simulink library "basic_THB"  (R2016b)
settings: Solver=ode45  StartTime=0.0  StopTime=10.0  RelTol=1e-3  EnableMultiTasking=on
undefined symbols (not defined in the file): Water
settings Model: Creator=lena.frank  LastModifiedBy=awohlfei
settings DataIOCC: LimitDataPoints=on  SaveFormat=Array  SignalLoggingSaveFormat=ModelDataLogs
settings OptimizationCC: ExpressionDepthLimit=2147483647  LifeSpan=inf
settings DebuggingCC: UnderspecifiedInitializationDetection=Classic  MergeDetectMultiDrivingBlocksExec=none  SolverPrmCheckMsg=warning  FcnCallInpInsideContextMsg=warning  StateNameClashWarn=warning  SFUnexpectedBacktrackingDiag=warning  SFNoUnconditionalDefaultTransitionDiag=warning  SFExecutionAtInitializationDiag=none
settings HardwareCC: ProdBitPerPointer=32  ProdBitPerSizeT=32  ProdBitPerPtrDiffT=32  ProdLargestAtomicFloat=None  ProdIntDivRoundTo=Undefined  ProdEndianess=Unspecified  ProdWordSize=32  ProdHWDeviceType=32-bit Generic
settings ModelReferenceCC: PropagateSignalLabelsOutOfModel=off
settings GRTTargetCC: TargetLangStandard=C89/C90 (ANSI)  GeneratePreprocessorConditionals=Disable all  CombineOutputUpdateFcns=off  GRTInterface=on
settings ConfigComp: CovMetricSettings=dw  CovHtmlReporting=on  CovSaveCumulativeToWorkspaceVar=on  CovSaveSingleToWorkspaceVar=on  CovExternalEMLEnable=off

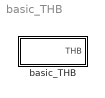
== system basic_THB ==
  basic_THB : Subsystem  InitFcn=load('THB.mat');  mask(basic THB){t=20, mdot=0, p=1e5, ID=Pressure Drop from Massflow, fluid=Water, mix=0, mix2=0, mix3=0, dia=0.02, hgt=0}
      mask prompts: t "temperature [°C]"; mdot "massflow [kg/s]"; p "pressure [Pa]"; ID "ID for pressure drop calculation"; mix "fluid mixture [0..1]"; mix2 "fluid mixture 2 [0..1]"; mix3 "fluid mixture 3 [0..1]"; dia "diameter [m]"; hgt "Static height in m"
      mask help:
      | Create a constant Thermo-Hydraulic-Vector.
      | Pressure drop calculation mode (defined by ID):
      |     1 ..  9999 no pressure drop (dp)
      | 10001 .. 19999 dp caused by flowrate
      | 20001 .. inf   dp by flowrate and static height
      mask Help: web(fullfile(path_carnot('help'),'basic_THB.html'),'-helpbrowser')
      mask TypeOptions t: const24/Value
      mask TypeOptions mdot: const25/Value
      mask TypeOptions p: const26/Value
      mask TypeOptions ID: const21/mID
      mask TypeOptions fluid: const27/fluid
      mask TypeOptions mix: const28/Value
      mask TypeOptions mix2: const2/Value
      mask TypeOptions mix3: const3/Value
      mask TypeOptions dia: const29/Value
      mask TypeOptions hgt: const1/Value

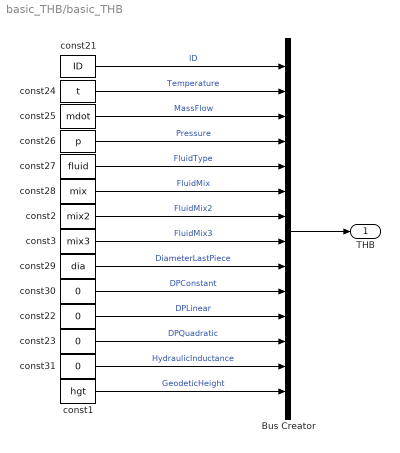
== system basic_THB/basic_THB ==
  Bus Creator : BusCreator  InitFcn=load THB.mat  Inputs=14  OutDataTypeStr=Bus: THB
  const1 : Constant  Value=hgt
  const2 : Constant  Value=mix2
  const21 : Constant  Value=ID  mask{mID=Pressure Drop from Massflow}
      mask prompts: mID "ID for pressure drop calculation"
      mask init:
      | ID = (mID-1)*10000+1;
      mask TypeOptions mID: No Pressure Drop | Pressure Drop from Massflow | Full Pressure Drop with Static Height
  const{22..23,30..31} (4 alike) : Constant  Value=0
  const24 : Constant  Value=t
  const25 : Constant  Value=mdot
  const26 : Constant  Value=p
  const27 : Constant  Value=fluid  mask{fluid=Water}
      mask TypeOptions fluid: Water | Air | Cotton Oil | Silicone Oil | Water-Glycol Mix | Tyfocor LS | Water (Constant 20°C) | Air (dry+ constant 20°C)
  const28 : Constant  Value=mix
  const29 : Constant  Value=dia
  const3 : Constant  Value=mix3
  THB : Outport
  wires:
  const3/1 -> Bus Creator/8  "FluidMix3"
  const2/1 -> Bus Creator/7  "FluidMix2"
  const1/1 -> Bus Creator/14  "GeodeticHeight"
  const31/1 -> Bus Creator/13  "HydraulicInductance"
  const23/1 -> Bus Creator/12  "DPQuadratic"
  const22/1 -> Bus Creator/11  "DPLinear"
  const29/1 -> Bus Creator/9  "DiameterLastPiece"
  const30/1 -> Bus Creator/10  "DPConstant"
  Bus Creator/1 -> THB/1
  const21/1 -> Bus Creator/1  "ID"
  const24/1 -> Bus Creator/2  "Temperature"
  const25/1 -> Bus Creator/3  "MassFlow"
  const26/1 -> Bus Creator/4  "Pressure"
  const27/1 -> Bus Creator/5  "FluidType"
  const28/1 -> Bus Creator/6  "FluidMix"
